simulink model "CanBusRagnar2020b"  (R2021b)
settings: Solver=VariableStepAuto  StartTime=0.0  StopTime=6  RelTol=1e-3
values from neighbouring files (symbols this model uses):
  F_mimo = -F_mimo    [SS_MIMO.m]    (also in controller_code.m = [-95.1662         0         0         0  -24.6981         0 ; workspace.mat = [-1.46285714286 0 0 0 0 -3.44816326531 0 0 0 0 -3.0563265306)
  L_mimo = -place(A',C',Desired_poles_obs)'    [SS_MIMO.m]    (also in workspace.mat = [-2 0 0 0 0 0 0 0 0 -1.85714285714 0 0 ... (64 elements, 8x8)
  sys_mimo = ss(A,B,C,0)    [SS_MIMO.m]
libraries: simulink_extras x6, truetime x6, dspsrcs4 x2
settings Model: Creator=mozzr  LastModifiedBy=krist
settings SolverCC: AlgebraicLoopSolver=TrustRegion

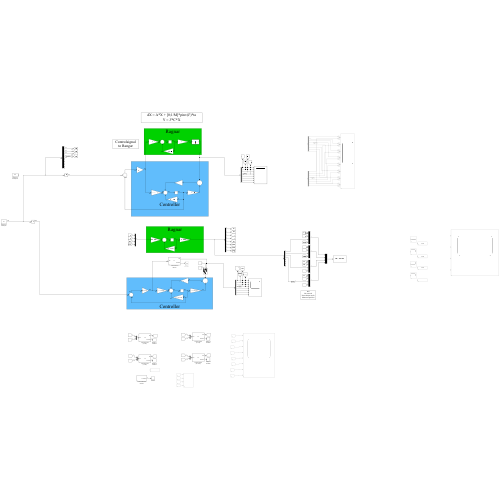
[thumbnail: Simulink's stored preview of the top-level diagram]
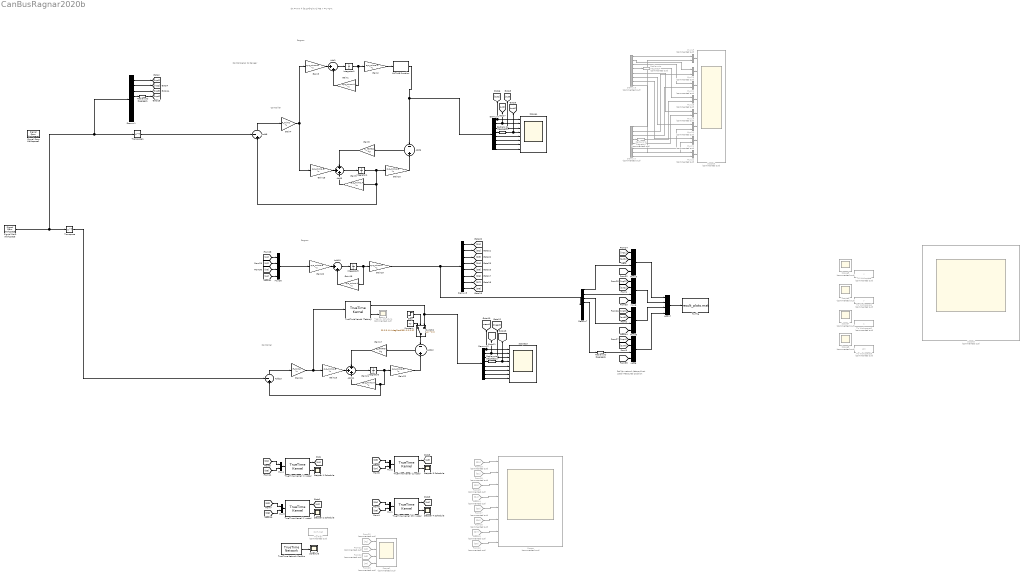
== system CanBusRagnar2020b ==
  note: Ragnar
  note: Controller
  note: Controller
  note: dX = A*X + [0;1/M]*pinv(J')*ta
      | Y = J'*C*X
  note: Controlsignal
      | to Rangar
  note: Ragnar
  note: Ref
      | No network
      | Network(not used)
      | Measured position
  Add1 : Sum  Inputs=|++
  Add10 : Sum  Inputs=|++
  Add11 : Sum  Inputs=+++
  Add12 : Sum  Inputs=-+
  Add13 : Sum  Inputs=-+|
  Add5 : Sum  Inputs=+++
  Add6 : Sum  Inputs=-+
  Add8 : Sum  Inputs=-+|
  Constant : Constant  Value=[0 0.5 -0.4 deg2rad(90) 0 0 0 0]'
  Demux{1,4,7..8,12} (5 alike) : Demux  Outputs=8
  Demux2 : Demux  Commented=on  Outputs=8
  Demux3 : Demux  Commented=on  Outputs=8
  From12 : From  Commented=on  GotoTag=O8
  From13 : From  Commented=on  GotoTag=O7
  From14 : From  Commented=on  GotoTag=O4
  From15 : From  Commented=on  GotoTag=O3
  From16 : From  Commented=on  GotoTag=O6
  From17 : From  Commented=on  GotoTag=O5
  From18 : From  Commented=on  GotoTag=O2
  From19 : From  Commented=on  GotoTag=O1
  From20 : From  Commented=on  GotoTag=A1
  From21 : From  Commented=on  GotoTag=A2
  From22 : From  Commented=on  GotoTag=A3
  From23 : From  Commented=on  GotoTag=A4
  Gain{1,9,18,21} (4 alike) : Gain  Gain=sys_mimo.A  Multiplication=Matrix(K*u)
  Gain{2,10,19,22} (4 alike) : Gain  Gain=sys_mimo.C  Multiplication=Matrix(K*u)
  Gain{3,15,20,23} (4 alike) : Gain  Gain=sys_mimo.B  Multiplication=Matrix(K*u)
  Gain16 : Gain  Gain=F_mimo  Multiplication=Matrix(K*u)
  Gain17 : Gain  Gain=L_mimo  Multiplication=Matrix(K*u)
  Gain4 : Gain  Gain=F_mimo  Multiplication=Matrix(K*u)
  Gain5 : Gain  Gain=L_mimo  Multiplication=Matrix(K*u)
  Integrator{1,4..6} (4 alike) : Integrator  InitialCondition=[0 0.5 -0.4 deg2rad(90) 0 0 0 0]'
  MATLAB Function : MATLAB Function  TreatAsAtomicUnit=on
  Mux{1..4} (4 alike) : Mux  Inputs=2
  Mux{5..6,15,17,26,35} (6 alike) : Mux
  Mux{18..25} (8 alike) : Mux  Commented=on  Inputs=2
  Radians to Degrees{1,3,6,11} (4 alike) : simulink_extras/Transformations/Radians to Degrees
  Radians to Degrees2 : simulink_extras/Transformations/Radians to Degrees  Commented=on
  Radians to Degrees4 : simulink_extras/Transformations/Radians to Degrees  Commented=on
  Schedule : Scope
  Scope : Scope  Commented=on  NumInputPorts=8
  Scope1 : Scope  Commented=on  NumInputPorts=4
  Scope13 : Scope  NumInputPorts=8
  Scope2 : Scope  Commented=on  NumInputPorts=4
  Scope3 : Scope  Commented=on  NumInputPorts=8
  Scope4 : Scope  NumInputPorts=8
  Scope{5..8} (4 alike) : Scope  Commented=on
  Signal From Workspace : dspsrcs4/Signal From Workspace  X=ref  Ts=1  nsamps=1  OutputAfterFinalValue=Holding final value  ignoreOrWarnInputAndFrameLengths=off  OutputFrames=off
  Signal From Workspace1 : dspsrcs4/Signal From Workspace  X=ref1  Ts=1  nsamps=1  OutputAfterFinalValue=Holding final value  ignoreOrWarnInputAndFrameLengths=off  OutputFrames=off
  Step : Step  Time=0.0025  Before=1  After=0  SampleTime=0
  Stepper 1 Schedule : Scope
  Stepper 2 Schedule : Scope
  Stepper 3 Schedule : Scope
  Stepper 4 Schedule : Scope
  Switch2 : Switch  Criteria=u2 ~= 0  Threshold=1
  Teensy Schedule : Scope  Commented=on
  To File : ToFile  Filename=result_plots.mat  SaveFormat=Timeseries
  To File1 : ToFile  Commented=on  Filename=NwT.mat  SaveFormat=Timeseries
  To Workspace : ToWorkspace  Commented=on  VariableName=x  SaveFormat=Timeseries  SampleTime=-1
  To Workspace1 : ToWorkspace  Commented=on  VariableName=y  SaveFormat=Timeseries  SampleTime=-1
  To Workspace2 : ToWorkspace  Commented=on  VariableName=z  SaveFormat=Timeseries  SampleTime=-1
  To Workspace3 : ToWorkspace  Commented=on  VariableName=phi  SaveFormat=Timeseries  SampleTime=-1
  Transpose : Math  Operator=transpose  SaturateOnIntegerOverflow=on
  Transpose1 : Math  Operator=transpose  SaturateOnIntegerOverflow=on
  TrueTime Kernel (Phi node) : truetime/TrueTime Kernel  sfun=nodePhi_init  args=[]  ninputsoutputs=[2 1]  ntriggers=0  trigtype=falling  nwnodenbr=[1 5]  clockoffsetdrift=[0 0]  schedoutput=on  battery=off  poweroutput=off  label=1: 5
  TrueTime Kernel (Teensy) : truetime/TrueTime Kernel  sfun=Teensy_init  args=[]  ninputsoutputs=[4 8]  ntriggers=0  trigtype=falling  nwnodenbr=[1 1]  clockoffsetdrift=[0 0]  schedoutput=on  battery=off  poweroutput=off  label=1: 1
  TrueTime Kernel (X node) : truetime/TrueTime Kernel  sfun=nodeX_init  args=[]  ninputsoutputs=[2 1]  ntriggers=0  trigtype=falling  nwnodenbr=[1 2]  clockoffsetdrift=[0 0]  schedoutput=on  battery=off  poweroutput=off  label=1: 2
  TrueTime Kernel (Y node) : truetime/TrueTime Kernel  sfun=nodeY_init  args=[]  ninputsoutputs=[2 1]  ntriggers=0  trigtype=falling  nwnodenbr=[1 3]  clockoffsetdrift=[0 0]  schedoutput=on  battery=off  poweroutput=off  label=1: 3
  TrueTime Kernel (Z node) : truetime/TrueTime Kernel  sfun=nodeZ_init  args=[]  ninputsoutputs=[2 1]  ntriggers=0  trigtype=falling  nwnodenbr=[1 4]  clockoffsetdrift=[0 0]  schedoutput=on  battery=off  poweroutput=off  label=1: 4
  TrueTime Network CanBus : truetime/TrueTime Network  nwtype=CSMA/AMP (CAN)  nwnbr=1  nnodes=5  rate=10000000  minsize=512  lossprob=0  seed=0  bandwidths=[0.5 0.5]  slotsize=512  schedule=[1 1 2]  memsize=80000  buftype=Common buffer  overflow=Retransmit  dynSchedule=0  miniSlotSize=0  NIT=0  QSortMode=FIFO  sync=0  irtSchedule=0  nrtLength=0  nodeGraph=0  scheduleoutput=on
  wires:
  TrueTime Kernel (Y node)/2 -> Stepper 2 Schedule/1
  TrueTime Kernel (X node)/2 -> Stepper 1 Schedule/1
  TrueTime Kernel (Phi node)/2 -> Stepper 4 Schedule/1
  TrueTime Kernel (Z node)/2 -> Stepper 3 Schedule/1
  TrueTime Kernel (Teensy)/2 -> Teensy Schedule/1
  TrueTime Network CanBus/1 -> Schedule/1
  TrueTime Kernel (X node)/1 -> [A1]
  TrueTime Kernel (Y node)/1 -> [A2]
  TrueTime Kernel (Phi node)/1 -> [A4]
  TrueTime Kernel (Z node)/1 -> [A3]
  Mux1/1 -> TrueTime Kernel (Phi node)/1
  [O4] -> Mux1/1
  [O8] -> Mux1/2
  [O3] -> Mux2/1
  [O7] -> Mux2/2
  Mux2/1 -> TrueTime Kernel (Z node)/1
  [O2] -> Mux3/1
  [O6] -> Mux3/2
  Mux3/1 -> TrueTime Kernel (Y node)/1
  [O1] -> Mux4/1
  [O5] -> Mux4/2
  Mux4/1 -> TrueTime Kernel (X node)/1
  From12/1 -> Scope/8
  From13/1 -> Scope/7
  From14/1 -> Scope/4
  From15/1 -> Scope/3
  From17/1 -> Scope/5
  From16/1 -> Scope/6
  From18/1 -> Scope/2
  From19/1 -> Scope/1
  From20/1 -> Scope1/1
  From21/1 -> Scope1/2
  From22/1 -> Scope1/3
  From23/1 -> Scope1/4
  Demux7/2 -> Mux6/3
  Radians to Degrees6/1 -> Mux5/3
  Demux7/1 -> Mux15/3
  Demux7/4 -> Radians to Degrees6/1
  Demux7/3 -> Mux35/3
  Mux5/1 -> Mux17/4
  Mux35/1 -> Mux17/3
  Mux6/1 -> Mux17/2
  Mux15/1 -> Mux17/1
  Demux1/4 -> Radians to Degrees1/1
  Demux1/1 -> [inp1]
  Demux1/2 -> [inp2]
  Demux1/3 -> [inp3]
  Radians to Degrees1/1 -> [inp4]
  [inp1] -> Mux15/1
  [inp2] -> Mux6/1
  [inp3] -> Mux35/1
  Mux17/1 -> To File/1
  Gain21/1 -> Add11/3
  Add13/1 -> Gain16/1
  Gain23/1 -> Add11/2
  Gain16/1 -> TrueTime Kernel (Teensy)/1, Gain23/1
  Integrator5/1 -> Gain18/1, Gain19/1
  Gain18/1 -> Add10/2
  Gain20/1 -> Add10/1
  Add11/1 -> Integrator6/1
  Add12/1 -> Gain17/1
  Gain22/1 -> Add12/2
  Add10/1 -> Integrator5/1
  Gain17/1 -> Add11/1
  Integrator6/1 -> Add13/2, Gain21/1, Gain22/1
  Gain5/1 -> Add5/1
  Integrator4/1 -> Gain10/1, Add8/2, Gain9/1
  Add8/1 -> Gain4/1
  Gain9/1 -> Add5/3
  Gain15/1 -> Add5/2
  Add5/1 -> Integrator4/1
  Gain4/1 -> Gain3/1, Gain15/1
  Add6/1 -> Gain5/1
  Mux23/1 -> Scope3/2
  Demux2/5 -> Mux19/2
  Demux2/8 -> Mux22/2
  Demux2/6 -> Mux20/2
  Mux18/1 -> Scope3/1
  Radians to Degrees4/1 -> Mux25/1
  Demux2/1 -> Mux18/2
  Demux2/7 -> Mux21/2
  Mux19/1 -> Scope3/5
  Demux3/8 -> Mux22/1
  Demux3/3 -> Mux24/1
  Mux24/1 -> Scope3/3
  Mux21/1 -> Scope3/7
  Demux3/1 -> Mux18/1
  Demux3/4 -> Radians to Degrees4/1
  Radians to Degrees2/1 -> Mux25/2
  Mux22/1 -> Scope3/8
  Demux3/7 -> Mux21/1
  Mux25/1 -> Scope3/4
  Demux2/3 -> Mux24/2
  Demux3/2 -> Mux23/1
  Mux20/1 -> Scope3/6
  Gain10/1 -> Add6/2
  Demux3/5 -> Mux19/1
  Demux2/2 -> Mux23/2
  Demux2/4 -> Radians to Degrees2/1
  Demux3/6 -> Mux20/1
  Demux8/8 -> [O8]
  Demux8/7 -> [O7]
  Demux8/4 -> [O4]
  Demux8/5 -> [O5]
  Demux8/3 -> [O3]
  Demux8/1 -> [O1]
  Demux8/2 -> [O2]
  Demux8/6 -> [O6]
  [A4] -> Mux26/4
  [A3] -> Mux26/3
  [A2] -> Mux26/2
  [A1] -> Mux26/1
  Mux26/1 -> Gain20/1
  Add1/1 -> Integrator1/1
  Gain1/1 -> Add1/2
  Integrator1/1 -> Gain1/1, Gain2/1
  Gain3/1 -> Add1/1
  Transpose/1 -> Add13/1
  Gain19/1 -> Demux7/1, Demux8/1
  Demux12/6 -> Scope13/6
  Demux12/4 -> Radians to Degrees11/1
  Demux12/1 -> Scope13/1, [meas1]
  Demux12/8 -> Scope13/8
  Demux12/5 -> Scope13/5
  Demux12/2 -> Scope13/2, [meas2]
  Demux12/3 -> Scope13/3, [meas3]
  Demux12/7 -> Scope13/7
  Step/1 -> Switch2/2
  Constant/1 -> Switch2/1
  Switch2/1 -> Add12/1
  TrueTime Kernel (Teensy)/1 -> Switch2/3, Demux12/1
  Signal From Workspace/1 -> Transpose1/1, Demux1/1, Transpose/1
  Transpose1/1 -> Add8/1
  [out1] -> Mux15/2
  [out2] -> Mux6/2
  [out3] -> Mux35/2
  [out4] -> Mux5/2
  [inp4] -> Mux5/1
  Radians to Degrees11/1 -> Scope13/4, [meas4]
  [meas4] -> Mux5/4
  [meas3] -> Mux35/4
  [meas2] -> Mux6/4
  [meas1] -> Mux15/4
  Radians to Degrees3/1 -> [out4], Scope4/4
  Demux4/4 -> Radians to Degrees3/1
  Demux4/5 -> Scope4/5
  Demux4/3 -> [out3], Scope4/3
  Demux4/2 -> [out2], Scope4/2
  Demux4/7 -> Scope4/7
  Demux4/6 -> Scope4/6
  Demux4/1 -> Scope4/1, [out1]
  Demux4/8 -> Scope4/8
  Gain2/1 -> MATLAB Function/1(u)
  MATLAB Function/1(y) -> Demux4/1, Add6/1

== matlab function CanBusRagnar2020b/MATLAB Function ==
  data: u input; y output
function y = fcn(u)
    TSRes = 0.0027;
    stepsCount = zeros(8,1);
    stepsCount([1:4],1) = round(u([1:4],1) ./ TSRes);
    stepsCount([1:4],1) = stepsCount([1:4],1) .* TSRes;
    y=u;
    y([1:4],1) = stepsCount([1:4],1);
end
